simulink model "INTERLOCK_DELAY_OLD"  (R2016a)
settings: Solver=FixedStepDiscrete  StartTime=0.0  StopTime=10.0  RelTol=1e-3
undefined symbols (not defined in the file): sigbuilder_block
libraries: simulink x6
settings Model: Creator=zedboard  LastModifiedBy=Wendel
settings OptimizationCC: BlockReduction=off  ConditionallyExecuteInputs=off  DefaultParameterBehavior=Inlined
settings DebuggingCC: AlgebraicLoopMsg=error
settings HardwareCC: ProdBitPerPointer=32  ProdLargestAtomicFloat=None  ProdIntDivRoundTo=Undefined  ProdEndianess=Unspecified  ProdWordSize=32  ProdHWDeviceType=ASIC/FPGA->ASIC/FPGA  ProdEqTarget=off

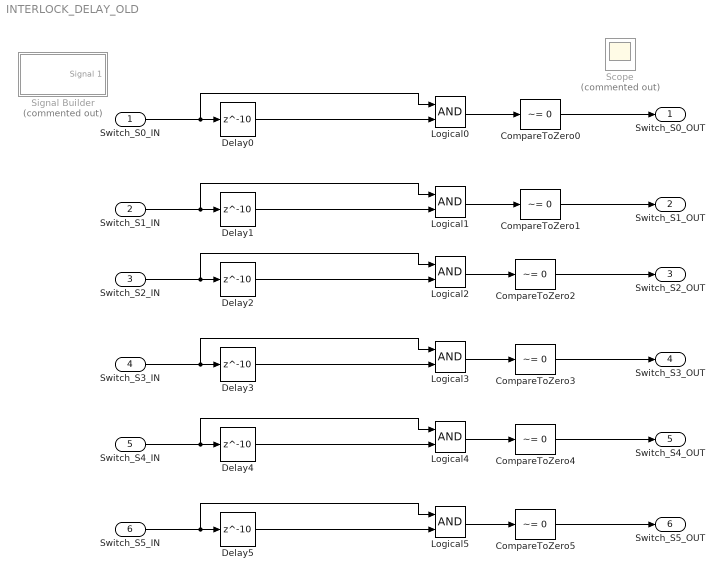
== system INTERLOCK_DELAY_OLD ==
  Switch_S0_IN : Inport  OutDataTypeStr=boolean
  Switch_S1_IN : Inport  Port=2  OutDataTypeStr=boolean
  Switch_S2_IN : Inport  Port=3  OutDataTypeStr=boolean
  Switch_S3_IN : Inport  Port=4  OutDataTypeStr=boolean
  Switch_S4_IN : Inport  Port=5  OutDataTypeStr=boolean
  Switch_S5_IN : Inport  Port=6  OutDataTypeStr=boolean
  CompareToZero{0..5} (6 alike) : simulink/Logic and Bit Operations/Compare To Zero  relop=~=  OutDataTypeStr=boolean
  Delay0 : Delay  DelayLength=10  InitialCondition=0  SampleTime=0.001
  Delay{1..5} (5 alike) : Delay  DelayLength=10  InitialCondition=0
  Logical{0..5} (6 alike) : Logic  AllPortsSameDT=off  OutDataTypeStr=boolean
  Scope : Scope  Commented=on  NumInputPorts=3
  Signal Builder : Subsystem  Tag=STV Subsys  Commented=on  LoadFcn=sigbuilder_block('load');  StartFcn=sigbuilder_block('start');  StopFcn=sigbuilder_block('stop');  ClipboardFcn=sigbuilder_block('clipboard');  mask(Sigbuilder block){}
      mask help: Simulink:masks:SigbuilderBlock_MD
      mask init:
      | if ~strcmp(get_param(bdroot(gcbh),'SimulationStatus'),'stopped') tuvar = sigbuilder_block('maskInit'); end
      settings: CopyFcn=sigbuilder_block('copy');  DeleteFcn=sigbuilder_block('delete');  ModelCloseFcn=sigbuilder_block('modelClose');  PreSaveFcn=sigbuilder_block('preSave');  PauseFcn=sigbuilder_block('pause');  ContinueFcn=sigbuilder_block('continue');  NameChangeFcn=sigbuilder_block('namechange');  OpenFcn=sigbuilder_block('open',[437.6 199.2 550.4 400 ]);  CloseFcn=sigbuilder_block('close');
      mask Display: plot(0, 0, 100, 100,[2, 2, 32, 32, 2], [68, 8, 8, 68, 68],[32, 2], [38, 38], [32, 19, 2],[53, 60, 44], [32, 17, 17, 2],[16, 16, 31, 31]);txt = getActiveGroup(gcbh);text(2, 100, txt,'verticalAlignment', 'top');
  Switch_S0_OUT : Outport
  Switch_S1_OUT : Outport  Port=2
  Switch_S2_OUT : Outport  Port=3
  Switch_S3_OUT : Outport  Port=4
  Switch_S4_OUT : Outport  Port=5
  Switch_S5_OUT : Outport  Port=6
  wires:
  Switch_S0_IN/1 -> Logical0/1, Delay0/1
  Delay0/1 -> Logical0/2
  Logical0/1 -> CompareToZero0/1
  CompareToZero0/1 -> Switch_S0_OUT/1
  Switch_S1_IN/1 -> Logical1/1, Delay1/1
  Delay1/1 -> Logical1/2
  Logical1/1 -> CompareToZero1/1
  CompareToZero1/1 -> Switch_S1_OUT/1
  Switch_S2_IN/1 -> Logical2/1, Delay2/1
  Delay2/1 -> Logical2/2
  Logical2/1 -> CompareToZero2/1
  CompareToZero2/1 -> Switch_S2_OUT/1
  Switch_S3_IN/1 -> Logical3/1, Delay3/1
  Delay3/1 -> Logical3/2
  Logical3/1 -> CompareToZero3/1
  CompareToZero3/1 -> Switch_S3_OUT/1
  Switch_S4_IN/1 -> Logical4/1, Delay4/1
  Delay4/1 -> Logical4/2
  Logical4/1 -> CompareToZero4/1
  CompareToZero4/1 -> Switch_S4_OUT/1
  Switch_S5_IN/1 -> Logical5/1, Delay5/1
  Delay5/1 -> Logical5/2
  Logical5/1 -> CompareToZero5/1
  CompareToZero5/1 -> Switch_S5_OUT/1

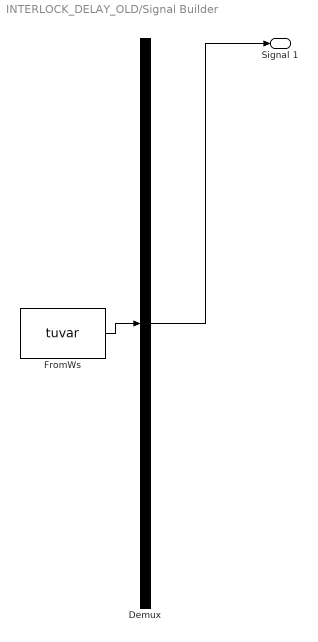
== system INTERLOCK_DELAY_OLD/Signal Builder ==
  Demux : Demux  Tag=STV Demux  Outputs=1
  FromWs : FromWorkspace  Tag=STV FromWs  VariableName=tuvar  SampleTime=0
      SigBuilderData=|
      | common.afterFinalStr = 'Extrapolate'
      | common.sampleTime = 0
      | dataSet.timeRange = [0 10]
      | dataSet.name = 'Group 1'
      | sbobj.Groups.Name = 'Group 1'
      | sbobj.Groups.Signals.Name = 'Signal 1'
      | sbobj.Groups.Signals.XData = [0 1.02 1.02 6 6 10]
      | sbobj.Groups.Signals.YData = [0 0 1 1 0 0]
  Signal 1 : Outport  Tag=STV Outport
  wires:
  Demux/1 -> Signal 1/1
  FromWs/1 -> Demux/1
